simulink model "DEEE_centre_tri"  (R2026a)
settings: Solver=VariableStepDiscrete  StopTime=T_sim
values from neighbouring files (symbols this model uses):
  dt = 0.25    [params_DEEE.m]
  MTBF = 120    [params_DEEE.m]
  MTBF_B1 = 80    [params_DEEE.m]    (also in scenarios_DEEE.m = MTBF_B1_scenarios(i))
  MTBF_B2 = 120    [params_DEEE.m]
  MTBF_Mag = 200    [params_DEEE.m]
  MTBF_Opt = 60    [params_DEEE.m]
  MTTR = 4    [params_DEEE.m]
  MTTR_B1 = 6    [params_DEEE.m]
  MTTR_B2 = 4    [params_DEEE.m]
  MTTR_Mag = 3    [params_DEEE.m]
  MTTR_Opt = 2    [params_DEEE.m]
  tau_capt_GEM = 0.94    [params_DEEE.m]
undefined symbols (not defined in the file or in its folder): m, n
(part 2 of 2)

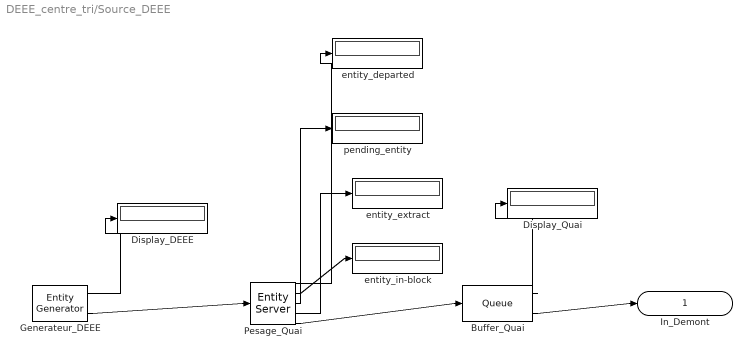
== system DEEE_centre_tri/Source_DEEE ==
  Buffer_Quai : Queue  InputPortMessageModes=m  OutputPortMessageModes=n,m  Capacity=inf  NumberEntitiesDeparted=on
      settings: OutputPortMap=o0,o5
  Display_DEEE : Display
  Display_Quai : Display
  Generateur_DEEE : EntityGenerator  OutputPortMessageModes=n,m  Period=dt  GenerateAction=|  AttributeName=categorie|masse|timestamp_entree|valorisable|tps_service|masse_fe|masse_nfe|masse_plastique|masse_verre|masse_autre|fraction_dominante|masse_recuperee|granulometrie|masse_Cu|masse_Au|masse_Ag|valeur_euro|dangereux|masse_bat|masse_Hg|nb_passages|route_depollution|grain_route|purete_Fe|rendement_Fe|pertes_Fe|purete_NFe|rendement_NFe|pertes_NFe|rendement_Plas|pertes_Plas|purete_Verre|rendement_Verre|pertes_Verre|purete_Plas|masse_Cu_init|masse_Au_init|masse_Ag_init|rendement_Cu|rendement_Au|rendement_Ag|energie_lixiv|energie_precip|energie_electro|energie_totale|conc_acide|pH_effluent|temp_cuve|eta_lixiv_reel|volume_effluent|energie_broyage|energie_tri|energie_separation|energie_totale_process|chaleur_recuperee|energie_lixiv_nette|taux_recuperation  AttributeInitialValue=0|0|0|1|0|0|0|0|0|0|1|0|0|0|0|0|0|0|0|0|0|2|1|0|0|0|0|0|0|0|0|0|0|0|0|0|0|0|0|0|0|0|0|0|0|0|0|0|0|0|0|0|0|0|0|0|0  NumberEntitiesDeparted=on  EntityType=Structured  EntityTypeName=DEEE
      | %% 1. CATÉGORIE
      | fractions = [0.42, 0.28, 0.18, 0.12];
      | r = rand();
      | cumul = cumsum(fractions);
      | if     r <= cumul(1); entity.categorie = 1;
      | elseif r <= cumul(2); entity.categorie = 2;
      | elseif r <= cumul(3); entity.categorie = 3;
      | else;                 entity.categorie = 4;
      | end
      | cat = entity.categorie;  % validation de cat
      | 
      | %% 2. MASSE
      | mu    = [3.50, 1.10, 2.08, 1.79];
      | sigma = [0.40, 0.35, 0.30, 0.35];
      | masse_kg = exp(mu(cat) + sigma(cat)*randn());
      | entity.masse = max(masse_kg, 0.5) / 1000;
      | 
      | %% 3. COMPOSITION MATIÈRE 
      | compo = [0.45, 0.12, 0.20, 0.00, 0.23;
      |          0.15, 0.25, 0.35, 0.00, 0.25;
      |          0.10, 0.18, 0.20, 0.30, 0.22;
      |          0.20, 0.30, 0.20, 0.05, 0.25];
      | 
      | entity.masse_fe        = entity.masse * compo(cat,1);
      | entity.masse_nfe       = entity.masse * compo(cat,2);
      | entity.masse_plastique = entity.masse * compo(cat,3);
      | entity.masse_verre     = entity.masse * compo(cat,4);
      | entity.masse_autre     = entity.masse * compo(cat,5);
      | 
      | %% 4. FRACTION DOMINANTE
      | fracs = [entity.masse_fe, entity.masse_nfe, ...
      |          entity.masse_plastique, entity.masse_verre, ...
      |          entity.masse_autre];
      | [~, entity.fraction_dominante] = max(fracs);
      | 
      | %%5. MÉTAUX PRÉCIEUX
      | metaux = [12.0,  0.8,  40.0;
      |           18.0,  3.5, 180.0;
      |           15.0,  8.0, 250.0;
      |           28.0, 12.0, 350.0];
      | 
      | masse_Cu_total = entity.masse * metaux(cat,1) / 1000;
      | masse_Au_total = entity.masse * metaux(cat,2);
      | masse_Ag_total = entity.masse * metaux(cat,3);
      | 
      | poids_nfe   = entity.masse_nfe   / entity.masse;
      | poids_autre = entity.masse_autre / entity.masse;
      | poids_total = poids_nfe + poids_autre;
      | 
      | if poids_total > 0
      |     entity.masse_Cu = masse_Cu_total * ...
      |         (0.70*poids_nfe + 0.25*poids_autre) / poids_total;
      |     entity.masse_Au = masse_Au_total * ...
      |         (0.70*poids_nfe + 0.25*poids_autre) / poids_total;
      |     entity.masse_Ag = masse_Ag_total * ...
      |         (0.70*poids_nfe + 0.25*poids_autre) / poids_total;
      | else
      |     entity.masse_Cu = masse_Cu_total * 0.05;
      |     entity.masse_Au = masse_Au_total * 0.05;
      |     entity.masse_Ag = masse_Ag_total * 0.05;
      | end
      | 
      | entity.valeur_euro = entity.masse_Cu * 8.5 + ...
      |                      entity.masse_Au  * 60.0 + ...
      |                      entity.masse_Ag  * 0.8;
      | 
      | %% 6. INITIALISATION
      | entity.valorisable       = 1;
      | entity.tps_service       = 0;
      | entity.masse_recuperee   = 0;
      | entity.granulometrie     = 0;
      | entity.dangereux         = 0;
      | entity.masse_bat         = 0;
      | entity.masse_Hg          = 0;
      | entity.route_depollution = 2; %sain par défaut
      | entity.nb_passages       = 0;
      | entity.grain_route       = 1;
      | 
      | % Sécurité—forcer attributs critiques valides
      | entity.categorie = max(1, min(4, round(entity.categorie)));
      | entity.valorisable = 1;
      | entity.grain_route = 1;
      | entity.route_depollution = 2;
      | entity.tps_service = 0.01;
      | % Sauvegarde des masses métaux précieux initiales
      | entity.masse_Cu_init = entity.masse_Cu;
      | entity.masse_Au_init = entity.masse_Au;
      | entity.masse_Ag_init = entity.masse_Ag;
      settings: OutputPortMap=o0,o3
  Pesage_Quai : EntityServer  InputPortMessageModes=m  OutputPortMessageModes=n,n,n,n,m  Capacity=50  ServiceTimeValue=0.001  NumberEntitiesDeparted=on  NumberEntitiesInBlock=on  PendingEntityPresentInBlock=on  NumEntitiesExtracted=on
      settings: OutputPortMap=o0,o1,o2,o12,o9
  entity_departed : Display
  entity_extract : Display
  entity_in-block : Display
  pending_entity : Display
  In_Demont : Outport
  wires:
  Generateur_DEEE/2 -> Pesage_Quai/1
  Pesage_Quai/5 -> Buffer_Quai/1
  Buffer_Quai/2 -> In_Demont/1
  Generateur_DEEE/1 -> Display_DEEE/1
  Buffer_Quai/1 -> Display_Quai/1
  Pesage_Quai/1 -> entity_departed/1
  Pesage_Quai/2 -> entity_in-block/1
  Pesage_Quai/3 -> pending_entity/1
  Pesage_Quai/4 -> entity_extract/1

== stateflow chart DEEE_centre_tri/SF_Magnetique ==
  state En_Service
    entry: disponible = 1;
    capacite = 10;
    t_panne = 0;
    t_maint = 0;
    t_panne_prochaine = -MTBF_eq * log(rand() + 0.0001);
    during: t_service = t_service + dt;
    T_total = t_service + t_panne + t_maint;
    if T_total > 0
    disponibilite = t_service / T_total;
    OEE_equip = disponibilite * performance * qualite;
    end
  state En_Panne
    entry: disponible = 0;
    capacite = 0;
    during: t_panne = t_panne + dt;
    T_total = t_service + t_panne + t_maint;
    if T_total > 0
    disponibilite = t_service / T_total;
    OEE_equip = disponibilite * performance * qualite;
    end
  state Maintenance
    entry: disponible = 0;
    capacite = 0;
    during: t_maint = t_maint + dt;
    T_total = t_service + t_panne + t_maint;
    if T_total > 0
    disponibilite = t_service / T_total;
    OEE_equip = disponibilite * performance * qualite;
    end
  (default) -> En_Service
  En_Service -> En_Panne : [t_service >= t_panne_prochaine]
  En_Panne -> Maintenance : [true]
  Maintenance -> En_Service : [t_maint >= MTTR_eq]
  data: t_service local =0; t_panne local =0; t_maint local =0; T_total local =0; t_panne_prochaine local =0; capacite output =10; disponible output =1; disponibilite output =1; OEE_equip output =0; MTBF_eq input; MTTR_eq input; dt input; performance input; qualite input

== stateflow chart DEEE_centre_tri/SF_Optique ==
  state En_Service
    entry: disponible = 1;
    capacite = 10;
    t_panne = 0;
    t_maint = 0;
    t_panne_prochaine = -MTBF_eq * log(rand() + 0.0001);
    during: t_service = t_service + dt;
    T_total = t_service + t_panne + t_maint;
    if T_total > 0
    disponibilite = t_service / T_total;
    OEE_equip = disponibilite * performance * qualite;
    end
  state En_Panne
    entry: disponible = 0;
    capacite = 0;
    during: t_panne = t_panne + dt;
    T_total = t_service + t_panne + t_maint;
    if T_total > 0
    disponibilite = t_service / T_total;
    OEE_equip = disponibilite * performance * qualite;
    end
  state Maintenance
    entry: disponible = 0;
    capacite = 0;
    during: t_maint = t_maint + dt;
    T_total = t_service + t_panne + t_maint;
    if T_total > 0
    disponibilite = t_service / T_total;
    OEE_equip = disponibilite * performance * qualite;
    end
  (default) -> En_Service
  En_Service -> En_Panne : [t_service >= t_panne_prochaine]
  En_Panne -> Maintenance : [true]
  Maintenance -> En_Service : [t_maint >= MTTR_eq]
  data: t_service local =0; t_panne local =0; t_maint local =0; T_total local =0; t_panne_prochaine local =0; capacite output =10; disponible output =1; disponibilite output =1; OEE_equip output =0; MTBF_eq input; MTTR_eq input; dt input; performance input; qualite input

== stateflow chart DEEE_centre_tri/SF_Broyeur2 ==
  state En_Service
    entry: disponible = 1;
    capacite = 10;
    t_panne = 0;
    t_maint = 0;
    t_panne_prochaine = -MTBF_eq * log(rand() + 0.0001);
    during: t_service = t_service + dt;
    T_total = t_service + t_panne + t_maint;
    if T_total > 0
    disponibilite = t_service / T_total;
    OEE_equip = disponibilite * performance * qualite;
    end
  state En_Panne
    entry: disponible = 0;
    capacite = 0;
    during: t_panne = t_panne + dt;
    T_total = t_service + t_panne + t_maint;
    if T_total > 0
    disponibilite = t_service / T_total;
    OEE_equip = disponibilite * performance * qualite;
    end
  state Maintenance
    entry: disponible = 0;
    capacite = 0;
    during: t_maint = t_maint + dt;
    T_total = t_service + t_panne + t_maint;
    if T_total > 0
    disponibilite = t_service / T_total;
    OEE_equip = disponibilite * performance * qualite;
    end
  (default) -> En_Service
  En_Service -> En_Panne : [t_service >= t_panne_prochaine]
  En_Panne -> Maintenance : [true]
  Maintenance -> En_Service : [t_maint >= MTTR_eq]
  data: t_service local =0; t_panne local =0; t_maint local =0; T_total local =0; t_panne_prochaine local =0; capacite output =10; disponible output =1; disponibilite output =1; OEE_equip output =0; MTBF_eq input; MTTR_eq input; dt input; performance input; qualite input

== stateflow chart DEEE_centre_tri/SF_Broyeur1 ==
  state En_Service
    entry: disponible = 1;
    capacite = 10;
    t_panne = 0;
    t_maint = 0;
    t_service = 0;
    T_total = 0;
    t_panne_prochaine = -MTBF_eq * log(rand() + 0.0001);
    during: t_service = t_service + dt;
    T_total = t_service + t_panne + t_maint;
    disponibilite = t_service / max(T_total, 0.0001);
    OEE_equip = disponibilite * performance * qualite;
    end
  state Maintenance
    entry: disponible = 0;
    capacite = 0;
    during: t_maint = t_maint + dt;
    T_total = t_service + t_panne + t_maint;
    disponibilite = t_service / max(T_total, 0.0001);
    OEE_equip = disponibilite * performance * qualite;
    end
  state En_Panne
    entry: disponible = 0;
    capacite = 0;
    during: t_panne = t_panne + dt;
    T_total = t_service + t_panne + t_maint;
    disponibilite = t_service / max(T_total, 0.0001);
    OEE_equip = disponibilite * performance * qualite;
    end
  (default) -> En_Service
  En_Service -> En_Panne : [t_service >= t_panne_prochaine]
  En_Panne -> Maintenance : [true]
  Maintenance -> En_Service : [t_maint >= MTTR_eq]
  data: t_service local =0; t_panne local =0; t_maint local =0; T_total local =0; t_panne_prochaine local =0; capacite output =10; disponible output =1; disponibilite output =1; OEE_equip output =0; MTBF_eq input; MTTR_eq input; dt input; performance input; qualite input

== stateflow chart DEEE_centre_tri/Pannes_Equipements ==
  state En_Service
    entry: disponible = 1;
    t_panne = 0;
    t_panne_prochaine = -MTBF * log(rand() + 0.0001);
    during: t_service = t_service + dt;
    T_total = t_service + t_panne + t_maint;
    if T_total > 0
    disponibilite = t_service / T_total;
    OEE = disponibilite * performance * qualite;
    end
  state En_Panne
    entry: disponible = 0;
    during: t_panne = t_panne + dt;
    T_total = t_service + t_panne + t_maint;
    if T_total > 0
    disponibilite = t_service / T_total;
    OEE = disponibilite * performance * qualite;
    end
  state Maintenance
    entry: disponible = 0;
    during: t_maint = t_maint + dt;
    T_total = t_service + t_panne + t_maint;
    if T_total > 0
    disponibilite = t_service / T_total;
    OEE = disponibilite * performance * qualite;
    end
  (default) -> En_Service
  En_Service -> En_Panne : [t_service >= t_panne_prochaine]
  En_Panne -> Maintenance : [true]
  Maintenance -> En_Service : [t_maint >= MTTR]
  data: dt input size=1; disponible output size=1 =1; t_service local size=1 =0; t_panne local size=1 =0; t_maint local size=1 =0; MTTR input size=1; OEE output size=1 =0; performance input size=1; T_total local size=1 =0; qualite input double size=1; t_panne_prochaine local size=1 =0; MTBF input; disponibilite output =1
